simulink model "Garcia_RA_Simulink_No2"  (R2023b)
settings: Solver=VariableStepAuto  StartTime=0.0  StopTime=20  RelTol=1e-3
values from neighbouring files (symbols this model uses):
  G_den = [A C E G I A]    [BAES_CSE_StepResponse_SecondOrder_UnderdampedSystem.m]    (also in BAES_CSE_StepResponse_SecondOrder_UnderdampedSystem_and_NonlinearSystemApproximation.m; Garcia_RA_MATLAB_No2.m = [b c d]; Lab2_StepResponse_FirstOrderSystem.m = [b c]; Lab2_StepResponse_ResonantSystem.m = [h i j k l m n o])
  G_num = [J H F D B]    [BAES_CSE_StepResponse_SecondOrder_UnderdampedSystem.m]    (also in BAES_CSE_StepResponse_SecondOrder_UnderdampedSystem_and_NonlinearSystemApproximation.m; Garcia_RA_MATLAB_No2.m = [a]; Lab2_StepResponse_FirstOrderSystem.m = [a]; Lab2_StepResponse_ResonantSystem.m = [a b c d e f g])
settings Model: Creator=ASUS  LastModifiedBy=ASUS

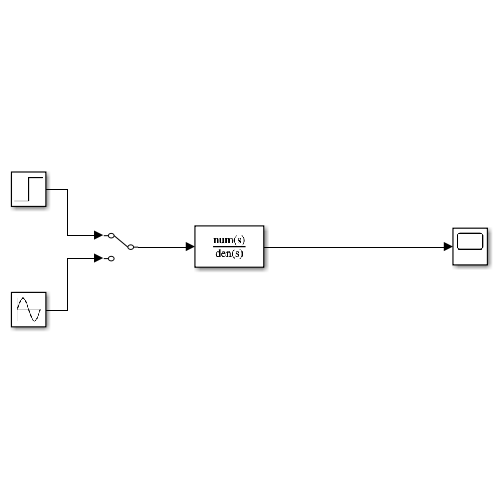
[thumbnail: Simulink's stored preview of the top-level diagram]
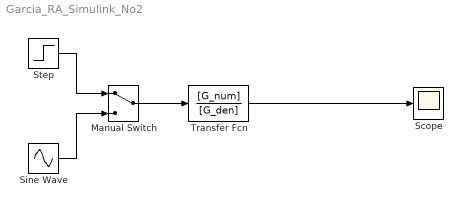
== system Garcia_RA_Simulink_No2 ==
  Manual Switch : ManualSwitch
  Scope : Scope
  Sine Wave : Sin  SampleTime=0
  Step : Step  Time=0  SampleTime=0
  Transfer Fcn : TransferFcn  Numerator=[G_num]  Denominator=[G_den]
  wires:
  Transfer Fcn/1 -> Scope/1
  Step/1 -> Manual Switch/1
  Sine Wave/1 -> Manual Switch/2
  Manual Switch/1 -> Transfer Fcn/1
